simulink model "HeldtModel2002"  (R2020b)
settings: Solver=ode45  StartTime=0.0  StopTime=60  MaxStep=stepsize_max  MinStep=stepsize_min  RelTol=1e-3
values from neighbouring files (symbols this model uses):
  C_a = 2.0    (= 2)    [HeldtModel2002startup.m]
  C_pa = 4.3    [HeldtModel2002startup.m]
  C_pv = 8.4    [HeldtModel2002startup.m]
  E_rv_dia = 1/C_rv_dia    (= 0.05)    [HeldtModel2002startup.m]
  E_rv_sys = 1/C_rv_sys    (= 0.833333333333)    [HeldtModel2002startup.m]
  freq = 2*pi*RR/60    (= 1.25663706144)    [HeldtModel2002startup.m]    (also in HeldtModel2004startup.m)
  P_th_bias = (P_th_high+P_th_low)/2    (= -5)    [HeldtModel2002startup.m]    (also in HeldtModel2004startup.m)
  R_inf = 3    [HeldtModel2002startup.m]
  R_kid1 = 4.1    [HeldtModel2002startup.m]
  R_ll1 = 3.6    [HeldtModel2002startup.m]
  R_lo = 0.006    [HeldtModel2002startup.m]
  R_p = 0.08    [HeldtModel2002startup.m]
  R_pv = 0.01    [HeldtModel2002startup.m]
  R_ro = 0.003    [HeldtModel2002startup.m]
  R_sp1 = 3.0    (= 3)    [HeldtModel2002startup.m]
  R_up1 = 3.9    [HeldtModel2002startup.m]
settings Model: Creator=sider  LastModifiedBy=sider

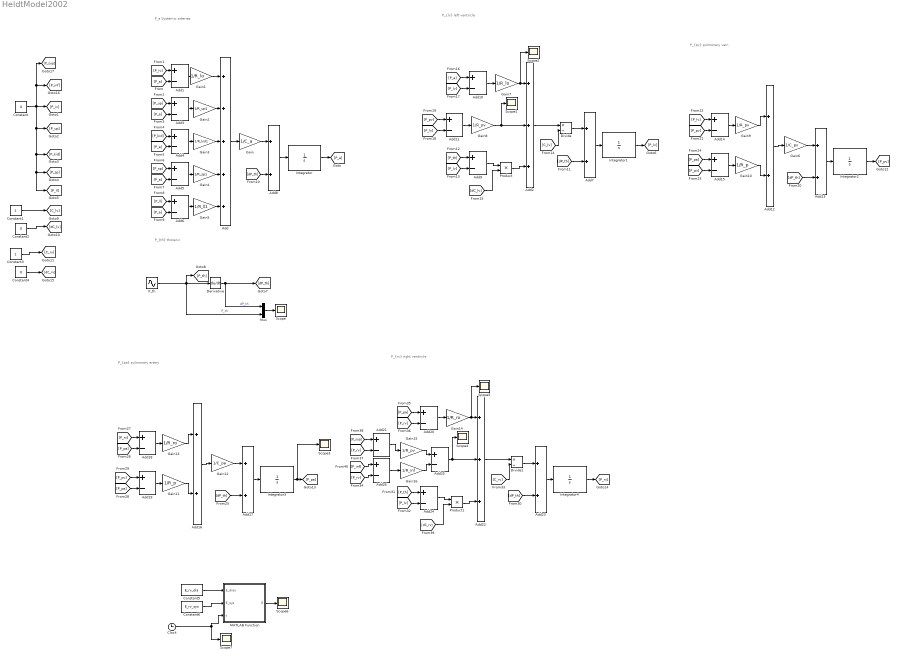
== system HeldtModel2002 ==
  note: P_a Systemic arteries
  note: P_{th} thoracic
  note: P_{lv} left ventricle
  note: P_{pv} pulmonary vein
  note: P_{pa} pulmonary artery
  note: P_{rv} right ventricle
  Add : Sum  Inputs=+++++
  Add{1,3..6,9..11,14..15,18..21,24..26} (17 alike) : Sum  Inputs=+-
  Add{7..8,12..13,16..17,23} (7 alike) : Sum
  Add2 : Sum  Inputs=+++
  Add22 : Sum  Inputs=+++
  Clock : Clock
  Constant : Constant  Value=0
  Constant1 : Constant
  Constant2 : Constant  Value=0
  Constant3 : Constant
  Constant4 : Constant  Value=0
  Constant5 : Constant  Value=E_rv_dia
  Constant6 : Constant  Value=E_rv_sys
  Derivative : Derivative
  Divide : Product  Inputs=*/
  Divide1 : Product  Inputs=*/
  Gain : Gain  Gain=1/C_a
  Gain1 : Gain  Gain=1/R_lo
  Gain10 : Gain  Gain=1/R_p
  Gain11 : Gain  Gain=1/R_p
  Gain12 : Gain  Gain=1/C_pa
  Gain13 : Gain  Gain=1/R_ro
  Gain14 : Gain  Gain=1/R_ro
  Gain15 : Gain  Gain=1/R_pv
  Gain16 : Gain  Gain=1/R_inf
  Gain2 : Gain  Gain=1/R_up1
  Gain3 : Gain  Gain=1/R_kid1
  Gain4 : Gain  Gain=1/R_sp1
  Gain5 : Gain  Gain=1/R_ll1
  Gain6 : Gain  Gain=1/C_pv
  Gain7 : Gain  Gain=1/R_lo
  Gain8 : Gain  Gain=1/R_pv
  Gain9 : Gain  Gain=1/R_pv
  Integrator{,1..4} (5 alike) : Integrator
  MATLAB Function : MATLAB Function  TreatAsAtomicUnit=on
  Mux : Mux  Inputs=2
  P_th : Sin  Bias=P_th_bias  Frequency=freq
  Product : Product
  Product1 : Product
  Scope{,1..7} (8 alike) : Scope
  wires:
  Add/1 -> Gain/1
  Add1/1 -> Gain1/1
  Gain1/1 -> Add/1
  [P_iv] -> Add1/1
  Constant/1 -> [P_sup], [P_inf], [P_ll], [P_sp], [P_kid], [P_up], [P_iv]
  Gain2/1 -> Add/2
  Add3/1 -> Gain2/1
  [P_a] -> Add1/2
  [P_up] -> Add3/1
  [P_a] -> Add3/2
  Gain3/1 -> Add/3
  [P_kid] -> Add4/1
  [P_a] -> Add4/2
  Add4/1 -> Gain3/1
  Gain4/1 -> Add/4
  Add5/1 -> Gain4/1
  [P_sp] -> Add5/1
  [P_a] -> Add5/2
  Gain5/1 -> Add/5
  Add6/1 -> Gain5/1
  [P_ll] -> Add6/1
  [P_a] -> Add6/2
  Integrator/1 -> [P_a]
  P_th/1 -> Mux/2, [P_th], Derivative/1  "P_th"
  Derivative/1 -> Mux/1, [dP_th]  "dP_th"
  Mux/1 -> Scope/1
  Gain/1 -> Add8/1
  [dP_th] -> Add8/2
  Add8/1 -> Integrator/1
  Add7/1 -> Integrator1/1
  [dP_th] -> Add7/2
  Integrator1/1 -> [P_lv]
  Divide/1 -> Add7/1
  Add2/1 -> Divide/1
  Gain7/1 -> Scope2/1, Add2/1
  Gain8/1 -> Scope1/1, Add2/2
  [P_th] -> Add9/1
  [P_lv] -> Add9/2
  Add9/1 -> Product/1
  Product/1 -> Add2/3
  [C_lv] -> Divide/2
  Constant1/1 -> [C_lv]
  Constant2/1 -> [dC_lv]
  [dC_lv] -> Product/2
  Add10/1 -> Gain7/1
  Add11/1 -> Gain8/1
  [P_a] -> Add10/1
  [P_lv] -> Add10/2
  [P_pv] -> Add11/1
  [P_lv] -> Add11/2
  Integrator2/1 -> [P_pv]
  Add13/1 -> Integrator2/1
  [dP_th] -> Add13/2
  Gain6/1 -> Add13/1
  Add12/1 -> Gain6/1
  Add14/1 -> Gain9/1
  [P_pv] -> Add14/2
  [P_lv] -> Add14/1
  Add15/1 -> Gain10/1
  [P_pv] -> Add15/2
  [P_pa] -> Add15/1
  Gain9/1 -> Add12/1
  Gain10/1 -> Add12/2
  Gain13/1 -> Add16/1
  [dP_th] -> Add17/2
  Integrator3/1 -> Scope3/1, [P_pa]
  [P_pa] -> Add18/2
  Add19/1 -> Gain11/1
  [P_pa] -> Add19/2
  Gain11/1 -> Add16/2
  [P_pv] -> Add19/1
  Add18/1 -> Gain13/1
  [P_rv] -> Add18/1
  Add16/1 -> Gain12/1
  Add17/1 -> Integrator3/1
  Gain12/1 -> Add17/1
  [dC_rv] -> Product1/2
  Add25/1 -> Scope4/1, Add22/2
  [P_pa] -> Add20/1
  Integrator4/1 -> [P_rv]
  Add23/1 -> Integrator4/1
  [dP_th] -> Add23/2
  Gain14/1 -> Scope5/1, Add22/1
  Add24/1 -> Product1/1
  Divide1/1 -> Add23/1
  [P_rv] -> Add20/2
  Product1/1 -> Add22/3
  Add20/1 -> Gain14/1
  Add22/1 -> Divide1/1
  [P_lv] -> Add24/2
  [C_rv] -> Divide1/2
  [P_th] -> Add24/1
  Constant3/1 -> [C_rv]
  Constant4/1 -> [dC_rv]
  [P_rv] -> Add21/2
  Add21/1 -> Gain15/1
  [P_sup] -> Add21/1
  Gain15/1 -> Add25/1
  Add26/1 -> Gain16/1
  [P_rv] -> Add26/2
  [P_inf] -> Add26/1
  Gain16/1 -> Add25/2
  Constant5/1 -> MATLAB Function/1(E_dias)
  Constant6/1 -> MATLAB Function/2(E_sys)
  Clock/1 -> MATLAB Function/3(t), Scope7/1
  MATLAB Function/1(E) -> Scope6/1

== matlab function HeldtModel2002/MATLAB Function ==
  data: E_dias input; E output; E_sys input; t input
function E = fcn(E_dias, E_sys, t)

t = mod(t,1);
T_n_m1 = 1;

%Bazett formula
T_s = 0.3*sqrt(T_n_m1);

if t > 0 && t < T_s

    E = E_dias + (E_sys+E_dias)*0.5*(1-cos(pi*t/(0.3*sqrt(T_n_m1))));
    
elseif t> T_s && t<= T_s*(3/2)
    E = E_dias + (E_sys+E_dias)*0.5*(1+cos((2*pi*(t-0.3*sqrt(T_n_m1)))/(0.3*sqrt(T_n_m1))));
else
    E = E_dias;
end
